simulink model "sensores"  (R2023b)
settings: Solver=VariableStepAuto  StartTime=0.0  StopTime=10.0  RelTol=1e-3
libraries: arduinolib x4, arduinosamdlib x4
settings Model: Creator=Usuario_UMA  LastModifiedBy=alumnos

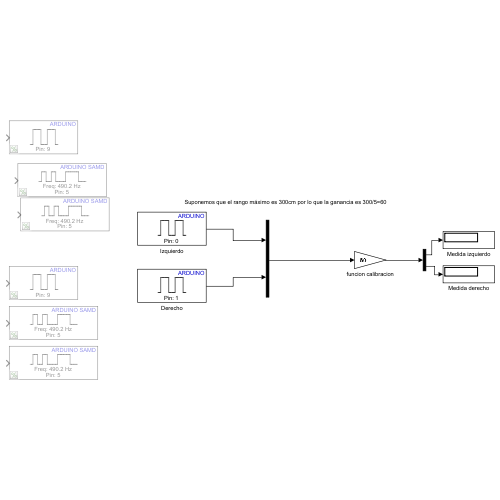
[thumbnail: Simulink's stored preview of the top-level diagram]
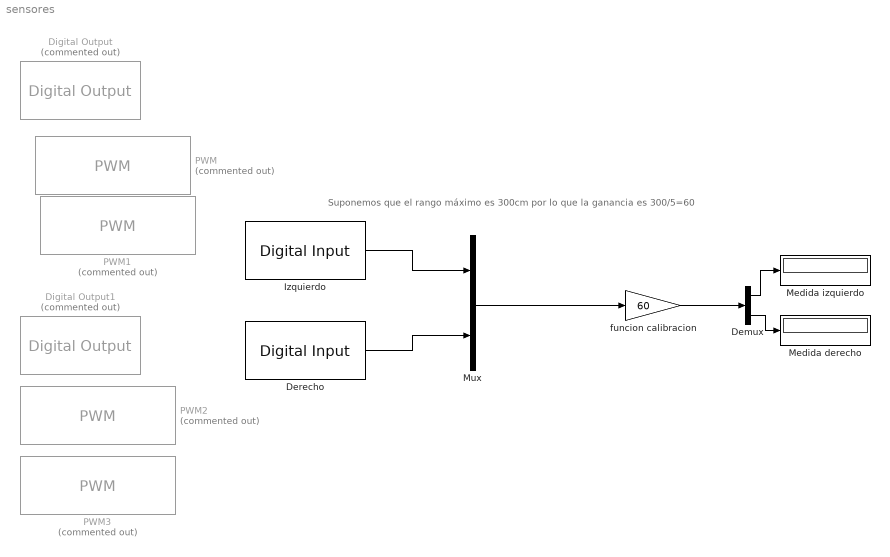
== system sensores ==
  note: Suponemos que el rango máximo es 300cm por lo que la ganancia es 300/5=60
  Demux : Demux  Outputs=2
  Derecho : arduinolib/Digital Input  pinNumber=1  mode=Default  Direction=input  SampleTime=0.1  blockPlatform=arduino
  Digital Output : arduinolib/Digital Output  Commented=on  pinNumber=9  Direction=output  blockPlatform=arduino
  Digital Output1 : arduinolib/Digital Output  Commented=on  pinNumber=9  Direction=output  blockPlatform=arduino
  Izquierdo : arduinolib/Digital Input  pinNumber=0  mode=Default  Direction=input  SampleTime=0.1  blockPlatform=arduino
  Medida derecho : Display
  Medida izquierdo : Display
  Mux : Mux  Inputs=2
  PWM{,1..3} (4 alike) : arduinosamdlib/PWM  Commented=on  pinNumber=5  desiredFrequency=490.2  achievableFrequency=490.2  wavegenMode=Dual-slope, interrupt/event at TOP (DSTOP)  EnableCompareMatchInterrupt=off  EnableOverflowInterrupt=on  InvertOutputPolarity=off
      settings: LibrarySourceBlock=arduinolib/PWM
  funcion calibracion : Gain  Gain=60
  wires:
  Izquierdo/1 -> Mux/1
  Derecho/1 -> Mux/2
  Mux/1 -> funcion calibracion/1
  funcion calibracion/1 -> Demux/1
  Demux/1 -> Medida izquierdo/1
  Demux/2 -> Medida derecho/1
